simulink model "PMSM_FOC_Compute"  (R2016b)
settings: Solver=FixedStepDiscrete  StartTime=0.0  StopTime=0.2  FixedStep=Params.h  RelTol=1e-3
undefined symbols (not defined in the file): Params
libraries: simulink x3
settings Model: DataTypeOverride=Double  MinMaxOverflowLogging=ForceOff  SimulationMode=processor-in-the-loop (pil)  Creator=Pascal  LastModifiedBy=Kevin
settings DataIOCC: LimitDataPoints=on  SaveFormat=Array
settings OptimizationCC: DefaultParameterBehavior=Inlined  LifeSpan=1
settings DebuggingCC: UnderspecifiedInitializationDetection=Classic  MergeDetectMultiDrivingBlocksExec=none  SolverPrmCheckMsg=warning  MultiTaskDSMMsg=none  AllowSymbolicDim=off  StateNameClashWarn=warning  SFUnexpectedBacktrackingDiag=warning  SFNoUnconditionalDefaultTransitionDiag=warning  SFExecutionAtInitializationDiag=none
settings HardwareCC: ProdBitPerPointer=32  ProdBitPerSizeT=32  ProdBitPerPtrDiffT=32  ProdLargestAtomicInteger=Integer  ProdWordSize=32  ProdHWDeviceType=STMicroelectronics->STM32 32-bit Cortex-M
settings ModelReferenceCC: PropagateSignalLabelsOutOfModel=off
settings RTWCC: SystemTargetFile=stm32.tlc  TemplateMakefile=stm32.tmf  Description=stm32 (Embedded Target)  GenerateReport=on  IncludeHyperlinkInReport=on  CreateSILPILBlock=PIL  CodeExecutionProfiling=on  CodeProfilingSaveOptions=AllData  GenerateCodeReplacementReport=on
settings CodeAppCC: IgnoreCustomStorageClasses=off  MaxIdLength=64  CustomSymbolStrType=$N$R$M  SimulinkBlockComments=off
settings STFCustomTargetCC: CodeReplacementLibrary=ARM CMSIS SIN COS  ParMdlRefBuildCompliant=on  IncludeMdlTerminateFcn=off  CombineOutputUpdateFcns=on  ERTCustomFileBanners=on  SupportContinuousTime=off  SupportNonInlinedSFcns=off  RemoveResetFunc=on  MATLABClassNameForMDSCustomization=Simulink.SoftwareTarget.ERTCustomization  GRTInterface=off  SystemTargetFile=stm32.tlc
settings ERTTargetCC: CodeReplacementLibrary=ARM CMSIS SIN COS  CompOptLevelCompliant=off  ConcurrentExecutionCompliant=off  IncludeMdlTerminateFcn=off  ERTFirstTimeCompliant=off  ModelStepFunctionPrototypeControlCompliant=off  CPPClassGenCompliant=off  UseToolchainInfoCompliant=off  ExtModeMexArgs=0,4,115200,10  ERTSrcFileBannerTemplate=sourceFileTemplate.cgt  ERTHdrFileBannerTemplate=sourceFileTemplate.cgt  ERTDataSrcFileTemplate=sourceFileTemplate.cgt  ERTDataHdrFileTemplate=sourceFileTemplate.cgt  ERTCustomFileTemplate=customRoutineProcess.tlc  ConvertIfToSwitch=off  SuppressUnreachableDefaultCases=off
settings ConfigComp: CovMetricSettings=dw  CovHtmlReporting=on  CovSaveCumulativeToWorkspaceVar=on  CovSaveSingleToWorkspaceVar=on  CovExternalEMLEnable=off  CovSFcnEnable=off

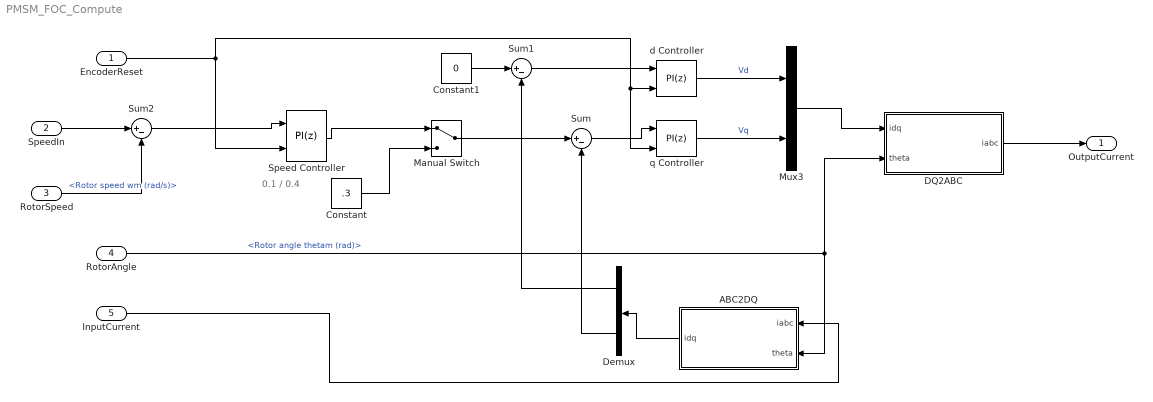
== system PMSM_FOC_Compute ==
  note: 0.1 / 0.4
  EncoderReset : Inport  OutDataTypeStr=boolean
  SpeedIn : Inport  Port=2  PortDimensions=1  Interpolate=off
  RotorSpeed : Inport  Port=3  PortDimensions=1  Interpolate=off
  RotorAngle : Inport  Port=4  OutDataTypeStr=single  PortDimensions=1
  InputCurrent : Inport  Port=5  OutDataTypeStr=single  PortDimensions=3
  ABC2DQ : MATLAB Function  TreatAsAtomicUnit=on
  Constant : Constant  Value=.3
  Constant1 : Constant  Value=0  OutDataTypeStr=single
  DQ2ABC : MATLAB Function  TreatAsAtomicUnit=on
  Demux : Demux  Outputs=2
  Manual Switch : ManualSwitch
  Mux3 : Mux  Inputs=2
  Speed Controller : simulink/Continuous/PID Controller  Controller=PI  TimeDomain=Discrete-time  SampleTime=Params.h  IntegratorMethod=Forward Euler  FilterMethod=Forward Euler  Form=Parallel  UseFilter=on  ControllerParametersSource=internal  P=0.0015  I=0.01  D=0.0005  N=100  InitialConditionSource=internal  InitialConditionForIntegrator=0  InitialConditionForFilter=0  ExternalReset=level  LimitOutput=on  UpperSaturationLimit=Params.Imax  LowerSaturationLimit=-Params.Imax  LinearizeAsGain=off  AntiWindupMode=back-calculation  Kb=0.015  TrackingMode=off  Kt=1  PParamMin=[]  PParamMax=[]  PParamDataTypeStr=single  IParamMin=[]  IParamMax=[]  IParamDataTypeStr=single  DParamMin=[]  DParamMax=[]  NParamMin=[]  NParamMax=[]  KbParamMin=[]  KbParamMax=[]  KbParamDataTypeStr=single  KtParamMin=[]  KtParamMax=[]  POutMin=[]  POutMax=[]  POutDataTypeStr=single  PGainOutDataTypeStr=single  PProdOutDataTypeStr=single  IOutMin=[]  IOutMax=[]  IOutDataTypeStr=single  IGainOutDataTypeStr=single  IProdOutDataTypeStr=single  DOutMin=[]  DOutMax=[]  NOutMin=[]  NOutMax=[]  KbOutMin=[]  KbOutMax=[]  KbOutDataTypeStr=single  KtOutMin=[]  KtOutMax=[]  IntegratorOutMin=[]  IntegratorOutMax=[]  IntegratorOutDataTypeStr=single  FilterOutMin=[]  FilterOutMax=[]  SumOutMin=[]  SumOutMax=[]  SumOutDataTypeStr=single  SumI1OutMin=[]  SumI1OutMax=[]  SumI1OutDataTypeStr=single  SumI2OutMin=[]  SumI2OutMax=[]  SumI2OutDataTypeStr=single  SumI3OutMin=[]  SumI3OutMax=[]  SumDOutMin=[]  SumDOutMax=[]  SumAccumDataTypeStr=single  SumI1AccumDataTypeStr=single  SumI2AccumDataTypeStr=single  SaturationOutMin=[]  SaturationOutMax=[]  SaturationOutDataTypeStr=single  IntegratorContinuousStateAttributes=''  IntegratorStateIdentifier=si  IntegratorStateMustResolveToSignalObject=off  IntegratorRTWStateStorageClass=Auto  FilterContinuousStateAttributes=''  FilterStateMustResolveToSignalObject=off  FilterRTWStateStorageClass=Auto  DifferentiatorICPrevScaledInput=0  DifferentiatorOutMin=[]  DifferentiatorOutMax=[]
  Sum : Sum  Inputs=|+-
  Sum1 : Sum  Inputs=|+-
  Sum2 : Sum  Inputs=|+-  InputSameDT=on
  d Controller : simulink/Continuous/PID Controller  Controller=PI  TimeDomain=Discrete-time  SampleTime=Params.h  IntegratorMethod=Forward Euler  FilterMethod=Forward Euler  Form=Parallel  UseFilter=on  ControllerParametersSource=internal  P=0  I=300  D=0.09  N=100  InitialConditionSource=internal  InitialConditionForIntegrator=0  InitialConditionForFilter=0  ExternalReset=level  LimitOutput=on  UpperSaturationLimit=Params.V  LowerSaturationLimit=-Params.V  LinearizeAsGain=off  AntiWindupMode=back-calculation  Kb=300  TrackingMode=off  Kt=1  PParamMin=[]  PParamMax=[]  PParamDataTypeStr=single  IParamMin=[]  IParamMax=[]  IParamDataTypeStr=single  DParamMin=[]  DParamMax=[]  NParamMin=[]  NParamMax=[]  KbParamMin=[]  KbParamMax=[]  KbParamDataTypeStr=single  KtParamMin=[]  KtParamMax=[]  POutMin=[]  POutMax=[]  POutDataTypeStr=single  PGainOutDataTypeStr=single  PProdOutDataTypeStr=single  IOutMin=[]  IOutMax=[]  IOutDataTypeStr=single  IGainOutDataTypeStr=single  IProdOutDataTypeStr=single  DOutMin=[]  DOutMax=[]  NOutMin=[]  NOutMax=[]  KbOutMin=[]  KbOutMax=[]  KbOutDataTypeStr=single  KtOutMin=[]  KtOutMax=[]  IntegratorOutMin=[]  IntegratorOutMax=[]  IntegratorOutDataTypeStr=single  FilterOutMin=[]  FilterOutMax=[]  SumOutMin=[]  SumOutMax=[]  SumOutDataTypeStr=single  SumI1OutMin=[]  SumI1OutMax=[]  SumI1OutDataTypeStr=single  SumI2OutMin=[]  SumI2OutMax=[]  SumI2OutDataTypeStr=single  SumI3OutMin=[]  SumI3OutMax=[]  SumDOutMin=[]  SumDOutMax=[]  SumAccumDataTypeStr=single  SumI1AccumDataTypeStr=single  SumI2AccumDataTypeStr=single  SaturationOutMin=[]  SaturationOutMax=[]  SaturationOutDataTypeStr=single  IntegratorContinuousStateAttributes=''  IntegratorStateIdentifier=di  IntegratorStateMustResolveToSignalObject=off  IntegratorRTWStateStorageClass=Auto  FilterContinuousStateAttributes=''  FilterStateMustResolveToSignalObject=off  FilterRTWStateStorageClass=Auto  DifferentiatorICPrevScaledInput=0  DifferentiatorOutMin=[]  DifferentiatorOutMax=[]
  q Controller : simulink/Continuous/PID Controller  Controller=PI  TimeDomain=Discrete-time  SampleTime=Params.h  IntegratorMethod=Forward Euler  FilterMethod=Forward Euler  Form=Parallel  UseFilter=on  ControllerParametersSource=internal  P=0  I=300  D=0.09  N=100  InitialConditionSource=internal  InitialConditionForIntegrator=0  InitialConditionForFilter=0  ExternalReset=level  LimitOutput=on  UpperSaturationLimit=Params.V  LowerSaturationLimit=-Params.V  LinearizeAsGain=off  AntiWindupMode=back-calculation  Kb=300  TrackingMode=off  Kt=1  PParamMin=[]  PParamMax=[]  PParamDataTypeStr=single  IParamMin=[]  IParamMax=[]  IParamDataTypeStr=single  DParamMin=[]  DParamMax=[]  NParamMin=[]  NParamMax=[]  KbParamMin=[]  KbParamMax=[]  KbParamDataTypeStr=single  KtParamMin=[]  KtParamMax=[]  POutMin=[]  POutMax=[]  POutDataTypeStr=single  PGainOutDataTypeStr=single  PProdOutDataTypeStr=single  IOutMin=[]  IOutMax=[]  IOutDataTypeStr=single  IGainOutDataTypeStr=single  IProdOutDataTypeStr=single  DOutMin=[]  DOutMax=[]  NOutMin=[]  NOutMax=[]  KbOutMin=[]  KbOutMax=[]  KbOutDataTypeStr=single  KtOutMin=[]  KtOutMax=[]  IntegratorOutMin=[]  IntegratorOutMax=[]  IntegratorOutDataTypeStr=single  FilterOutMin=[]  FilterOutMax=[]  SumOutMin=[]  SumOutMax=[]  SumOutDataTypeStr=single  SumI1OutMin=[]  SumI1OutMax=[]  SumI1OutDataTypeStr=single  SumI2OutMin=[]  SumI2OutMax=[]  SumI2OutDataTypeStr=single  SumI3OutMin=[]  SumI3OutMax=[]  SumDOutMin=[]  SumDOutMax=[]  SumAccumDataTypeStr=single  SumI1AccumDataTypeStr=single  SumI2AccumDataTypeStr=single  SaturationOutMin=[]  SaturationOutMax=[]  SaturationOutDataTypeStr=single  IntegratorContinuousStateAttributes=''  IntegratorStateIdentifier=qi  IntegratorStateMustResolveToSignalObject=off  IntegratorRTWStateStorageClass=Auto  FilterContinuousStateAttributes=''  FilterStateMustResolveToSignalObject=off  FilterRTWStateStorageClass=Auto  DifferentiatorICPrevScaledInput=0  DifferentiatorOutMin=[]  DifferentiatorOutMax=[]
  OutputCurrent : Outport  OutDataTypeStr=single
  wires:
  RotorAngle/1 -> ABC2DQ/2(theta), DQ2ABC/2(theta)  "<Rotor angle thetam (rad)>"
  RotorSpeed/1 -> Sum2/2  "<Rotor speed wm (rad/s)>"
  Sum/1 -> q Controller/1
  Constant1/1 -> Sum1/1
  Sum1/1 -> d Controller/1
  q Controller/1 -> Mux3/2  "Vq"
  d Controller/1 -> Mux3/1  "Vd"
  Manual Switch/1 -> Sum/1
  Speed Controller/1 -> Manual Switch/1
  Constant/1 -> Manual Switch/2
  Sum2/1 -> Speed Controller/1
  Mux3/1 -> DQ2ABC/1(idq)
  Demux/1 -> Sum1/2
  Demux/2 -> Sum/2
  ABC2DQ/1(idq) -> Demux/1
  DQ2ABC/1(iabc) -> OutputCurrent/1
  InputCurrent/1 -> ABC2DQ/1(iabc)
  SpeedIn/1 -> Sum2/1
  EncoderReset/1 -> d Controller/2, q Controller/2, Speed Controller/2

== matlab function PMSM_FOC_Compute/DQ2ABC ==
  data: iabc output; idq input; theta input
function iabc = ABC2DQ(idq,theta)

T = [cos(cast(theta,'single')) -sin(cast(theta,'single'));...
    cos(cast(theta-2*pi/3,'single'))  -sin(cast(theta-2*pi/3,'single'));...
    cos(cast(theta+2*pi/3,'single')) -sin(cast(theta+2*pi/3,'single'))];

iabc = T*idq;

== matlab function PMSM_FOC_Compute/ABC2DQ ==
  data: iabc input; idq output; theta input
function idq = ABC2DQ(iabc,theta)

T = 2/3 * [cos(cast(theta,'single')) cos(cast(theta-2*pi/3,'single')) cos(cast(theta+2*pi/3,'single'));...
    -sin(cast(theta,'single')) -sin(cast(theta-2*pi/3,'single')) -sin(cast(theta+2*pi/3,'single'))];

idq = T*iabc;
